simulink model "PhilippePetit_architecture"  (R2020b)
settings: Solver=VariableStepAuto  StartTime=0.0  StopTime=10.0  RelTol=1e-3
settings Model: Creator=nicol  LastModifiedBy=nicol

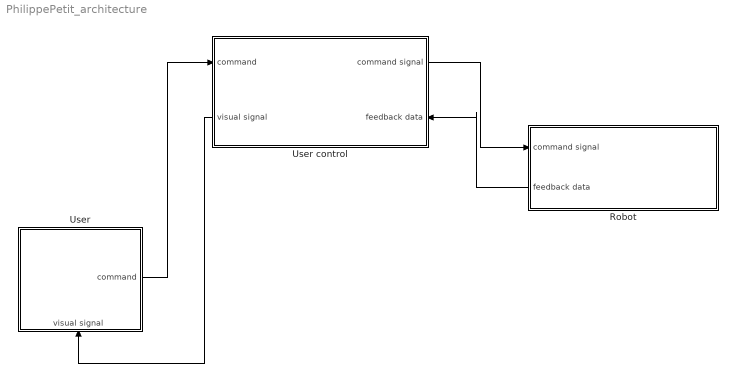
== system PhilippePetit_architecture ==
  Robot : Subsystem
      settings: PortSchema="{\"entries\":[{\"content\":{\"headerSize\":26,\"margin\":15,\"minimumSpacing\":25,\"sides\":[{\"content\":{\"connectorIds\":[\"In1\",\"Out1\"]},\"type\":\"ConnectorPlacement.EquallySpacedRectSide\",\"uuid\":\"a13b1b13-38f4-4b06-bb72-140aa99d31de\"},{\"content\":{\"connectorIds\":[],\"side\":\"RIGHT\"},\"type\":\"ConnectorPlacement.EquallySpacedRectSide\",\"uuid\":\"03928bee-4773-4998-99f8-4502b0986fa4\"},{\"content\":{\"connectorIds\":[],\"side\":\"TOP\"},\"type\":\"ConnectorPlacement.EquallySpacedRectSide\",\"uuid\":\"614edb4f-75a9-4b46-be23-a150b878b705\"},{\"content\":{\"connectorIds\":[],\"side\":\"BOTTOM\"},\"type\":\"ConnectorPlacement.EquallySpacedRectSide\",\"uuid\":\"73503f2b-8796-4b66-885d-2b8b1e679955\"},{\"content\":{\"connectorIds\":[],\"side\":\"HIDDEN\"},\"type\":\"ConnectorPlacement.EquallySpacedRectSide\",\"uuid\":\"9ce51372-9279-48e8-af61-c2921102bc5c\"}]},\"type\":\"ConnectorPlacement.EquallySpacedConnector\",\"uuid\":\"eab28fec-6cb4-4970-8796-7f8236b3d049\"}],\"packageUris\":[\"http://schema.mathworks.com/mf0/Connector/R2020b\"],\"version\":\"1.0\"}"
  User : Subsystem
      settings: PortSchema="{\"entries\":[{\"content\":{\"headerSize\":26,\"margin\":15,\"minimumSpacing\":25,\"sides\":[{\"content\":{\"connectorIds\":[]},\"type\":\"ConnectorPlacement.EquallySpacedRectSide\",\"uuid\":\"fe61efcc-83aa-4783-a816-baaa20b10315\"},{\"content\":{\"connectorIds\":[\"Out1\"],\"side\":\"RIGHT\"},\"type\":\"ConnectorPlacement.EquallySpacedRectSide\",\"uuid\":\"af858a2b-5332-46b9-9432-959710be5434\"},{\"content\":{\"connectorIds\":[],\"side\":\"TOP\"},\"type\":\"ConnectorPlacement.EquallySpacedRectSide\",\"uuid\":\"0d27328e-6c51-4811-958e-b304a9a2605e\"},{\"content\":{\"connectorIds\":[\"In1\"],\"side\":\"BOTTOM\"},\"type\":\"ConnectorPlacement.EquallySpacedRectSide\",\"uuid\":\"966ce028-5962-4a17-8d73-90c152cb0045\"},{\"content\":{\"connectorIds\":[],\"side\":\"HIDDEN\"},\"type\":\"ConnectorPlacement.EquallySpacedRectSide\",\"uuid\":\"1191bd8a-d3b3-41e0-ab93-51888f24952b\"}]},\"type\":\"ConnectorPlacement.EquallySpacedConnector\",\"uuid\":\"d4b5a27a-45d4-44c0-bb5f-ae7473592f44\"}],\"packageUris\":[\"http://schema.mathworks.com/mf0/Connector/R2020b\"],\"version\":\"1.0\"}"
  User control : Subsystem
      settings: PortSchema="{\"entries\":[{\"content\":{\"headerSize\":26,\"margin\":15,\"minimumSpacing\":25,\"sides\":[{\"content\":{\"connectorIds\":[\"In1\",\"Out1\"]},\"type\":\"ConnectorPlacement.EquallySpacedRectSide\",\"uuid\":\"a13b1b13-38f4-4b06-bb72-140aa99d31de\"},{\"content\":{\"connectorIds\":[\"Out2\",\"In2\"],\"side\":\"RIGHT\"},\"type\":\"ConnectorPlacement.EquallySpacedRectSide\",\"uuid\":\"03928bee-4773-4998-99f8-4502b0986fa4\"},{\"content\":{\"connectorIds\":[],\"side\":\"TOP\"},\"type\":\"ConnectorPlacement.EquallySpacedRectSide\",\"uuid\":\"614edb4f-75a9-4b46-be23-a150b878b705\"},{\"content\":{\"connectorIds\":[],\"side\":\"HIDDEN\"},\"type\":\"ConnectorPlacement.EquallySpacedRectSide\",\"uuid\":\"9ce51372-9279-48e8-af61-c2921102bc5c\"}]},\"type\":\"ConnectorPlacement.EquallySpacedConnector\",\"uuid\":\"eab28fec-6cb4-4970-8796-7f8236b3d049\"}],\"packageUris\":[\"http://schema.mathworks.com/mf0/Connector/R2020b\"],\"version\":\"1.0\"}"
  wires:
  User/1(command) -> User control/1(command)
  User control/1(visual signal) -> User/1(visual signal)
  User control/2(command signal) -> Robot/1(" command signal")
  Robot/1(feedback data) -> User control/2(feedback data)

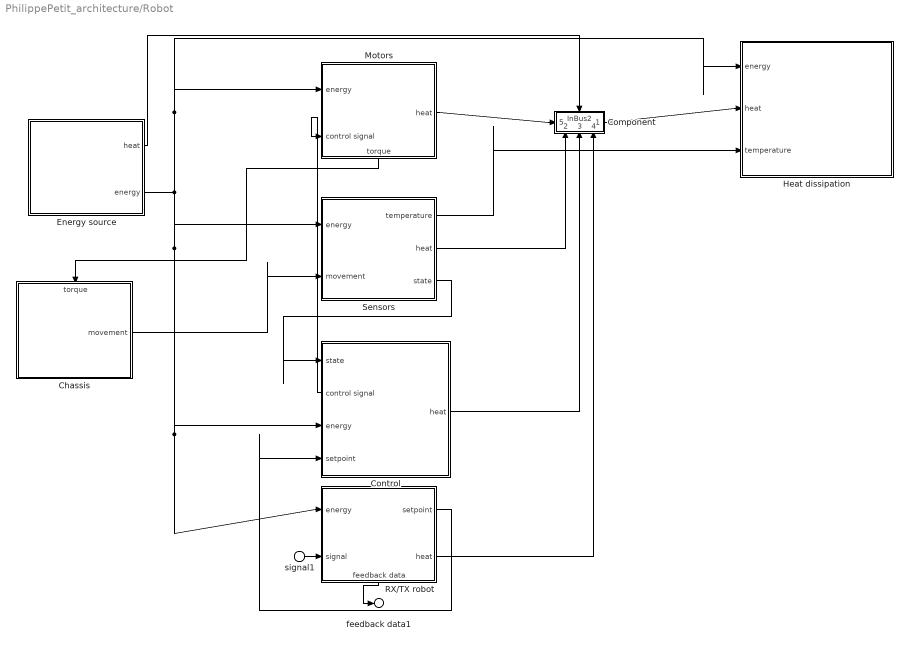
== system PhilippePetit_architecture/Robot ==
  " signal1" : Inport  PortName=command signal
  Chassis : Subsystem
      settings: PortSchema="{\"entries\":[{\"content\":{\"headerSize\":26,\"margin\":15,\"minimumSpacing\":25,\"sides\":[{\"content\":{\"connectorIds\":[]},\"type\":\"ConnectorPlacement.EquallySpacedRectSide\",\"uuid\":\"fe61efcc-83aa-4783-a816-baaa20b10315\"},{\"content\":{\"connectorIds\":[\"Out1\"],\"side\":\"RIGHT\"},\"type\":\"ConnectorPlacement.EquallySpacedRectSide\",\"uuid\":\"af858a2b-5332-46b9-9432-959710be5434\"},{\"content\":{\"connectorIds\":[\"In1\"],\"side\":\"TOP\"},\"type\":\"ConnectorPlacement.EquallySpacedRectSide\",\"uuid\":\"0d27328e-6c51-4811-958e-b304a9a2605e\"},{\"content\":{\"connectorIds\":[],\"side\":\"HIDDEN\"},\"type\":\"ConnectorPlacement.EquallySpacedRectSide\",\"uuid\":\"1191bd8a-d3b3-41e0-ab93-51888f24952b\"}]},\"type\":\"ConnectorPlacement.EquallySpacedConnector\",\"uuid\":\"d4b5a27a-45d4-44c0-bb5f-ae7473592f44\"}],\"packageUris\":[\"http://schema.mathworks.com/mf0/Connector/R2020b\"],\"version\":\"1.0\"}"
  Component : Subsystem
      settings: PortSchema="{\"entries\":[{\"content\":{\"margin\":10,\"minimumSpacing\":15,\"sides\":[{\"content\":{\"connectorIds\":[\"In5\"]},\"type\":\"ConnectorPlacement.EquallySpacedRectSide\",\"uuid\":\"fe61efcc-83aa-4783-a816-baaa20b10315\"},{\"content\":{\"connectorIds\":[\"Out1\"],\"side\":\"RIGHT\"},\"type\":\"ConnectorPlacement.EquallySpacedRectSide\",\"uuid\":\"af858a2b-5332-46b9-9432-959710be5434\"},{\"content\":{\"connectorIds\":[\"In1\"],\"side\":\"TOP\"},\"type\":\"ConnectorPlacement.EquallySpacedRectSide\",\"uuid\":\"0d27328e-6c51-4811-958e-b304a9a2605e\"},{\"content\":{\"connectorIds\":[\"In2\",\"In3\",\"In4\"],\"side\":\"BOTTOM\"},\"type\":\"ConnectorPlacement.EquallySpacedRectSide\",\"uuid\":\"543f712e-d5c5-44b2-9db3-03ae61feada7\"},{\"content\":{\"connectorIds\":[],\"side\":\"HIDDEN\"},\"type\":\"ConnectorPlacement.EquallySpacedRectSide\",\"uuid\":\"1191bd8a-d3b3-41e0-ab93-51888f24952b\"}]},\"type\":\"ConnectorPlacement.EquallySpacedConnector\",\"uuid\":\"d4b5a27a-45d4-44c0-bb5f-ae7473592f44\"}],\"packageUris\":[\"http://schema.mathworks.com/mf0/Connector/R2020b\"],\"version\":\"1.0\"}"
  Control : Subsystem
      settings: PortSchema="{\"entries\":[{\"content\":{\"headerSize\":26,\"margin\":15,\"minimumSpacing\":25,\"sides\":[{\"content\":{\"connectorIds\":[\"In1\",\"Out1\",\"In3\",\"In2\"]},\"type\":\"ConnectorPlacement.EquallySpacedRectSide\",\"uuid\":\"fe61efcc-83aa-4783-a816-baaa20b10315\"},{\"content\":{\"connectorIds\":[\"Out2\"],\"side\":\"RIGHT\"},\"type\":\"ConnectorPlacement.EquallySpacedRectSide\",\"uuid\":\"af858a2b-5332-46b9-9432-959710be5434\"},{\"content\":{\"connectorIds\":[],\"side\":\"TOP\"},\"type\":\"ConnectorPlacement.EquallySpacedRectSide\",\"uuid\":\"0d27328e-6c51-4811-958e-b304a9a2605e\"},{\"content\":{\"connectorIds\":[],\"side\":\"HIDDEN\"},\"type\":\"ConnectorPlacement.EquallySpacedRectSide\",\"uuid\":\"1191bd8a-d3b3-41e0-ab93-51888f24952b\"}]},\"type\":\"ConnectorPlacement.EquallySpacedConnector\",\"uuid\":\"d4b5a27a-45d4-44c0-bb5f-ae7473592f44\"}],\"packageUris\":[\"http://schema.mathworks.com/mf0/Connector/R2020b\"],\"version\":\"1.0\"}"
  Energy source : Subsystem
      settings: PortSchema="{\"entries\":[{\"content\":{\"headerSize\":26,\"margin\":15,\"minimumSpacing\":25,\"sides\":[{\"content\":{\"connectorIds\":[]},\"type\":\"ConnectorPlacement.EquallySpacedRectSide\",\"uuid\":\"fe61efcc-83aa-4783-a816-baaa20b10315\"},{\"content\":{\"connectorIds\":[\"Out1\",\"Out2\"],\"side\":\"RIGHT\"},\"type\":\"ConnectorPlacement.EquallySpacedRectSide\",\"uuid\":\"af858a2b-5332-46b9-9432-959710be5434\"},{\"content\":{\"connectorIds\":[],\"side\":\"TOP\"},\"type\":\"ConnectorPlacement.EquallySpacedRectSide\",\"uuid\":\"0d27328e-6c51-4811-958e-b304a9a2605e\"},{\"content\":{\"connectorIds\":[],\"side\":\"HIDDEN\"},\"type\":\"ConnectorPlacement.EquallySpacedRectSide\",\"uuid\":\"1191bd8a-d3b3-41e0-ab93-51888f24952b\"}]},\"type\":\"ConnectorPlacement.EquallySpacedConnector\",\"uuid\":\"d4b5a27a-45d4-44c0-bb5f-ae7473592f44\"}],\"packageUris\":[\"http://schema.mathworks.com/mf0/Connector/R2020b\"],\"version\":\"1.0\"}"
  Heat dissipation : Subsystem
      settings: PortSchema="{\"entries\":[{\"content\":{\"headerSize\":26,\"margin\":15,\"minimumSpacing\":25,\"sides\":[{\"content\":{\"connectorIds\":[\"In1\",\"In2\",\"In3\"]},\"type\":\"ConnectorPlacement.EquallySpacedRectSide\",\"uuid\":\"fe61efcc-83aa-4783-a816-baaa20b10315\"},{\"content\":{\"connectorIds\":[],\"side\":\"RIGHT\"},\"type\":\"ConnectorPlacement.EquallySpacedRectSide\",\"uuid\":\"af858a2b-5332-46b9-9432-959710be5434\"},{\"content\":{\"connectorIds\":[],\"side\":\"TOP\"},\"type\":\"ConnectorPlacement.EquallySpacedRectSide\",\"uuid\":\"0d27328e-6c51-4811-958e-b304a9a2605e\"},{\"content\":{\"connectorIds\":[],\"side\":\"HIDDEN\"},\"type\":\"ConnectorPlacement.EquallySpacedRectSide\",\"uuid\":\"1191bd8a-d3b3-41e0-ab93-51888f24952b\"}]},\"type\":\"ConnectorPlacement.EquallySpacedConnector\",\"uuid\":\"d4b5a27a-45d4-44c0-bb5f-ae7473592f44\"}],\"packageUris\":[\"http://schema.mathworks.com/mf0/Connector/R2020b\"],\"version\":\"1.0\"}"
  Motors : Subsystem
      settings: PortSchema="{\"entries\":[{\"content\":{\"headerSize\":26,\"margin\":15,\"minimumSpacing\":25,\"sides\":[{\"content\":{\"connectorIds\":[\"In1\",\"In2\"]},\"type\":\"ConnectorPlacement.EquallySpacedRectSide\",\"uuid\":\"fe61efcc-83aa-4783-a816-baaa20b10315\"},{\"content\":{\"connectorIds\":[\"Out2\"],\"side\":\"RIGHT\"},\"type\":\"ConnectorPlacement.EquallySpacedRectSide\",\"uuid\":\"af858a2b-5332-46b9-9432-959710be5434\"},{\"content\":{\"connectorIds\":[],\"side\":\"TOP\"},\"type\":\"ConnectorPlacement.EquallySpacedRectSide\",\"uuid\":\"0d27328e-6c51-4811-958e-b304a9a2605e\"},{\"content\":{\"connectorIds\":[\"Out1\"],\"side\":\"BOTTOM\"},\"type\":\"ConnectorPlacement.EquallySpacedRectSide\",\"uuid\":\"ab8045d5-2f64-4f7d-896e-5133e5fbee7e\"},{\"content\":{\"connectorIds\":[],\"side\":\"HIDDEN\"},\"type\":\"ConnectorPlacement.EquallySpacedRectSide\",\"uuid\":\"1191bd8a-d3b3-41e0-ab93-51888f24952b\"}]},\"type\":\"ConnectorPlacement.EquallySpacedConnector\",\"uuid\":\"d4b5a27a-45d4-44c0-bb5f-ae7473592f44\"}],\"packageUris\":[\"http://schema.mathworks.com/mf0/Connector/R2020b\"],\"version\":\"1.0\"}"
  RX/TX robot : Subsystem
      settings: PortSchema="{\"entries\":[{\"content\":{\"headerSize\":26,\"margin\":15,\"minimumSpacing\":25,\"sides\":[{\"content\":{\"connectorIds\":[\"In2\",\"In1\"]},\"type\":\"ConnectorPlacement.EquallySpacedRectSide\",\"uuid\":\"fe61efcc-83aa-4783-a816-baaa20b10315\"},{\"content\":{\"connectorIds\":[\"Out2\",\"Out3\"],\"side\":\"RIGHT\"},\"type\":\"ConnectorPlacement.EquallySpacedRectSide\",\"uuid\":\"af858a2b-5332-46b9-9432-959710be5434\"},{\"content\":{\"connectorIds\":[],\"side\":\"TOP\"},\"type\":\"ConnectorPlacement.EquallySpacedRectSide\",\"uuid\":\"0d27328e-6c51-4811-958e-b304a9a2605e\"},{\"content\":{\"connectorIds\":[\"Out1\"],\"side\":\"BOTTOM\"},\"type\":\"ConnectorPlacement.EquallySpacedRectSide\",\"uuid\":\"3b3053d7-3574-47a1-96ff-38e328b25c8b\"},{\"content\":{\"connectorIds\":[],\"side\":\"HIDDEN\"},\"type\":\"ConnectorPlacement.EquallySpacedRectSide\",\"uuid\":\"1191bd8a-d3b3-41e0-ab93-51888f24952b\"}]},\"type\":\"ConnectorPlacement.EquallySpacedConnector\",\"uuid\":\"d4b5a27a-45d4-44c0-bb5f-ae7473592f44\"}],\"packageUris\":[\"http://schema.mathworks.com/mf0/Connector/R2020b\"],\"version\":\"1.0\"}"
  Sensors : Subsystem
      settings: PortSchema="{\"entries\":[{\"content\":{\"headerSize\":26,\"margin\":15,\"minimumSpacing\":25,\"sides\":[{\"content\":{\"connectorIds\":[\"In1\",\"In2\"]},\"type\":\"ConnectorPlacement.EquallySpacedRectSide\",\"uuid\":\"fe61efcc-83aa-4783-a816-baaa20b10315\"},{\"content\":{\"connectorIds\":[\"Out1\",\"Out2\",\"Out3\"],\"side\":\"RIGHT\"},\"type\":\"ConnectorPlacement.EquallySpacedRectSide\",\"uuid\":\"af858a2b-5332-46b9-9432-959710be5434\"},{\"content\":{\"connectorIds\":[],\"side\":\"TOP\"},\"type\":\"ConnectorPlacement.EquallySpacedRectSide\",\"uuid\":\"0d27328e-6c51-4811-958e-b304a9a2605e\"},{\"content\":{\"connectorIds\":[],\"side\":\"HIDDEN\"},\"type\":\"ConnectorPlacement.EquallySpacedRectSide\",\"uuid\":\"1191bd8a-d3b3-41e0-ab93-51888f24952b\"}]},\"type\":\"ConnectorPlacement.EquallySpacedConnector\",\"uuid\":\"d4b5a27a-45d4-44c0-bb5f-ae7473592f44\"}],\"packageUris\":[\"http://schema.mathworks.com/mf0/Connector/R2020b\"],\"version\":\"1.0\"}"
  feedback data1 : Outport  PortName=feedback data
  wires:
  Control/2(heat) -> Component/3(InBus1)
  Energy source/2(energy) -> Heat dissipation/1(energy), Motors/1(energy), RX/TX robot/2(energy), Control/3(energy), Sensors/1(energy)
  Sensors/2(heat) -> Component/2(InBus)
  Sensors/3(state) -> Control/1(state)
  Sensors/1(temperature) -> Heat dissipation/3(temperature)
  RX/TX robot/1(feedback data) -> feedback data1/1
  RX/TX robot/2(setpoint) -> Control/2(setpoint)
  Component/1(tot heat) -> Heat dissipation/2(heat)
  RX/TX robot/3(heat) -> Component/4(heat)
  Motors/2(heat) -> Component/5(heat1)
  " signal1"/1 -> RX/TX robot/1(" signal")
  Energy source/1(heat) -> Component/1(InBus2)
  Control/1(control signal) -> Motors/2(control signal)
  Motors/1(torque) -> Chassis/1(torque)
  Chassis/1(movement) -> Sensors/2(movement)

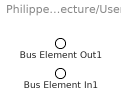
== system PhilippePetit_architecture/User ==
  Bus Element In1 : Inport  PortName=visual signal
  Bus Element Out1 : Outport  PortName=command

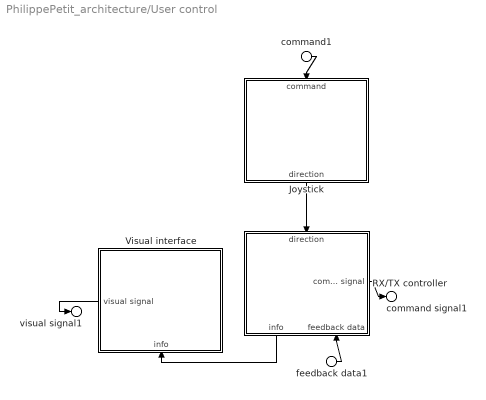
== system PhilippePetit_architecture/User control ==
  command1 : Inport  PortName=command
  feedback data1 : Inport  Port=2  PortName=feedback data
  Joystick : Subsystem
      settings: PortSchema="{\"entries\":[{\"content\":{\"headerSize\":26,\"margin\":15,\"minimumSpacing\":25,\"sides\":[{\"content\":{\"connectorIds\":[]},\"type\":\"ConnectorPlacement.EquallySpacedRectSide\",\"uuid\":\"fe61efcc-83aa-4783-a816-baaa20b10315\"},{\"content\":{\"connectorIds\":[],\"side\":\"RIGHT\"},\"type\":\"ConnectorPlacement.EquallySpacedRectSide\",\"uuid\":\"af858a2b-5332-46b9-9432-959710be5434\"},{\"content\":{\"connectorIds\":[\"In1\"],\"side\":\"TOP\"},\"type\":\"ConnectorPlacement.EquallySpacedRectSide\",\"uuid\":\"0d27328e-6c51-4811-958e-b304a9a2605e\"},{\"content\":{\"connectorIds\":[\"Out1\"],\"side\":\"BOTTOM\"},\"type\":\"ConnectorPlacement.EquallySpacedRectSide\",\"uuid\":\"2fc8f7ae-d563-416e-94db-7c5ffa9122e4\"},{\"content\":{\"connectorIds\":[],\"side\":\"HIDDEN\"},\"type\":\"ConnectorPlacement.EquallySpacedRectSide\",\"uuid\":\"1191bd8a-d3b3-41e0-ab93-51888f24952b\"}]},\"type\":\"ConnectorPlacement.EquallySpacedConnector\",\"uuid\":\"d4b5a27a-45d4-44c0-bb5f-ae7473592f44\"}],\"packageUris\":[\"http://schema.mathworks.com/mf0/Connector/R2020b\"],\"version\":\"1.0\"}"
  RX/TX controller : Subsystem
      settings: PortSchema="{\"entries\":[{\"content\":{\"headerSize\":26,\"margin\":15,\"minimumSpacing\":25,\"sides\":[{\"content\":{\"connectorIds\":[]},\"type\":\"ConnectorPlacement.EquallySpacedRectSide\",\"uuid\":\"fe61efcc-83aa-4783-a816-baaa20b10315\"},{\"content\":{\"connectorIds\":[\"Out2\"],\"side\":\"RIGHT\"},\"type\":\"ConnectorPlacement.EquallySpacedRectSide\",\"uuid\":\"af858a2b-5332-46b9-9432-959710be5434\"},{\"content\":{\"connectorIds\":[\"In2\"],\"side\":\"TOP\"},\"type\":\"ConnectorPlacement.EquallySpacedRectSide\",\"uuid\":\"0d27328e-6c51-4811-958e-b304a9a2605e\"},{\"content\":{\"connectorIds\":[\"Out1\",\"In1\"],\"side\":\"BOTTOM\"},\"type\":\"ConnectorPlacement.EquallySpacedRectSide\",\"uuid\":\"e34f4db2-095e-4c46-8f72-d51fa938d794\"},{\"content\":{\"connectorIds\":[],\"side\":\"HIDDEN\"},\"type\":\"ConnectorPlacement.EquallySpacedRectSide\",\"uuid\":\"1191bd8a-d3b3-41e0-ab93-51888f24952b\"}]},\"type\":\"ConnectorPlacement.EquallySpacedConnector\",\"uuid\":\"d4b5a27a-45d4-44c0-bb5f-ae7473592f44\"}],\"packageUris\":[\"http://schema.mathworks.com/mf0/Connector/R2020b\"],\"version\":\"1.0\"}"
  Visual interface : Subsystem
      settings: PortSchema="{\"entries\":[{\"content\":{\"headerSize\":26,\"margin\":15,\"minimumSpacing\":25,\"sides\":[{\"content\":{\"connectorIds\":[\"Out1\"]},\"type\":\"ConnectorPlacement.EquallySpacedRectSide\",\"uuid\":\"fe61efcc-83aa-4783-a816-baaa20b10315\"},{\"content\":{\"connectorIds\":[],\"side\":\"RIGHT\"},\"type\":\"ConnectorPlacement.EquallySpacedRectSide\",\"uuid\":\"af858a2b-5332-46b9-9432-959710be5434\"},{\"content\":{\"connectorIds\":[],\"side\":\"TOP\"},\"type\":\"ConnectorPlacement.EquallySpacedRectSide\",\"uuid\":\"0d27328e-6c51-4811-958e-b304a9a2605e\"},{\"content\":{\"connectorIds\":[\"In1\"],\"side\":\"BOTTOM\"},\"type\":\"ConnectorPlacement.EquallySpacedRectSide\",\"uuid\":\"5a0afe0c-1d89-46be-b1ab-40f5f276f1ed\"},{\"content\":{\"connectorIds\":[],\"side\":\"HIDDEN\"},\"type\":\"ConnectorPlacement.EquallySpacedRectSide\",\"uuid\":\"1191bd8a-d3b3-41e0-ab93-51888f24952b\"}]},\"type\":\"ConnectorPlacement.EquallySpacedConnector\",\"uuid\":\"d4b5a27a-45d4-44c0-bb5f-ae7473592f44\"}],\"packageUris\":[\"http://schema.mathworks.com/mf0/Connector/R2020b\"],\"version\":\"1.0\"}"
  visual signal1 : Outport  PortName=visual signal
  command signal1 : Outport  Port=2  PortName=command signal
  wires:
  RX/TX controller/2(command signal) -> command signal1/1
  Joystick/1(direction) -> RX/TX controller/2(direction)
  feedback data1/1 -> RX/TX controller/1(feedback data)
  command1/1 -> Joystick/1(command)
  RX/TX controller/1(info) -> Visual interface/1(info)
  Visual interface/1(visual signal) -> visual signal1/1

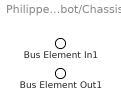
== system PhilippePetit_architecture/Robot/Chassis ==
  Bus Element In1 : Inport  PortName=torque
  Bus Element Out1 : Outport  PortName=movement

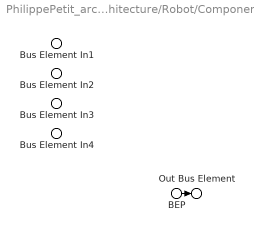
== system PhilippePetit_architecture/Robot/Component ==
  Bus Element In4 : Inport  PortName=InBus2
  Bus Element In2 : Inport  Port=2  PortName=InBus
  Bus Element In3 : Inport  Port=3  PortName=InBus1
  Bus Element In1 : Inport  Port=4  PortName=heat
  BEP : Inport  Port=5  PortName=heat1
  Out Bus Element : Outport  PortName=tot heat
  wires:
  BEP/1 -> Out Bus Element/1

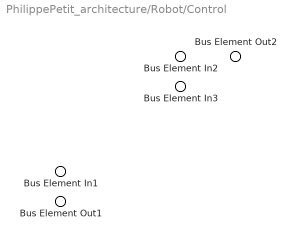
== system PhilippePetit_architecture/Robot/Control ==
  Bus Element In3 : Inport  PortName=state
  Bus Element In2 : Inport  Port=2  PortName=setpoint
  Bus Element In1 : Inport  Port=3  PortName=energy
  Bus Element Out2 : Outport  PortName=control signal
  Bus Element Out1 : Outport  Port=2  PortName=heat

== system PhilippePetit_architecture/Robot/Energy source ==
  Bus Element Out2 : Outport  PortName=heat
  Bus Element Out1 : Outport  Port=2  PortName=energy

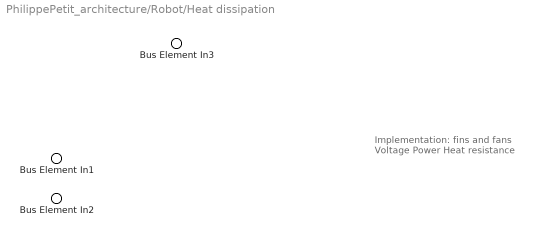
== system PhilippePetit_architecture/Robot/Heat dissipation ==
  note: Implementation: fins and fans
      | Voltage
      | Power
      | Heat resistance
  Bus Element In3 : Inport  PortName=energy
  Bus Element In1 : Inport  Port=2  PortName=heat
  Bus Element In2 : Inport  Port=3  PortName=temperature

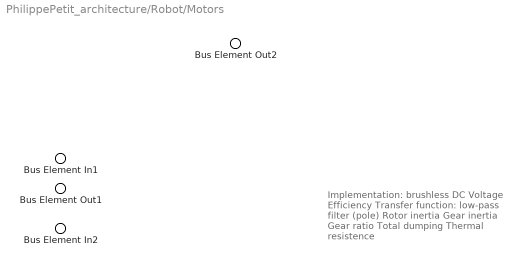
== system PhilippePetit_architecture/Robot/Motors ==
  note: Implementation: brushless DC
      | Voltage
      | Efficiency
      | Transfer function: low-pass filter (pole)
      | Rotor inertia
      | Gear inertia
      | Gear ratio
      | Total dumping
      | Thermal resistence
  Bus Element In1 : Inport  PortName=energy
  Bus Element In2 : Inport  Port=2  PortName=control signal
  Bus Element Out2 : Outport  PortName=torque
  Bus Element Out1 : Outport  Port=2  PortName=heat

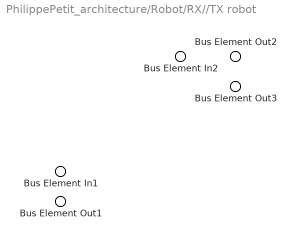
== system PhilippePetit_architecture/Robot/RX//TX robot ==
  Bus Element In2 : Inport  PortName=signal
  Bus Element In1 : Inport  Port=2  PortName=energy
  Bus Element Out3 : Outport  PortName=feedback data
  Bus Element Out2 : Outport  Port=2  PortName=setpoint
  Bus Element Out1 : Outport  Port=3  PortName=heat

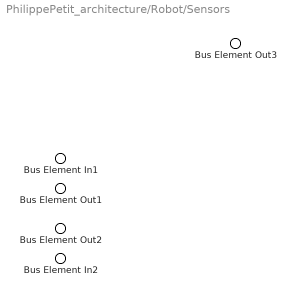
== system PhilippePetit_architecture/Robot/Sensors ==
  Bus Element In1 : Inport  PortName=energy
  Bus Element In2 : Inport  Port=2  PortName=movement
  Bus Element Out3 : Outport  PortName=temperature
  Bus Element Out1 : Outport  Port=2  PortName=heat
  Bus Element Out2 : Outport  Port=3  PortName=state

== system PhilippePetit_architecture/User control/Joystick ==
  Bus Element In1 : Inport  PortName=command
  Bus Element Out1 : Outport  PortName=direction

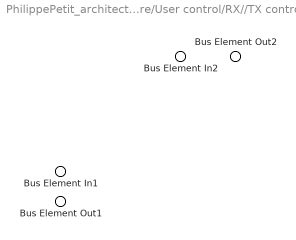
== system PhilippePetit_architecture/User control/RX//TX controller ==
  Bus Element In2 : Inport  PortName=feedback data
  Bus Element In1 : Inport  Port=2  PortName=direction
  Bus Element Out2 : Outport  PortName=info
  Bus Element Out1 : Outport  Port=2  PortName=command signal

== system PhilippePetit_architecture/User control/Visual interface ==
  Bus Element In1 : Inport  PortName=info
  Bus Element Out1 : Outport  PortName=visual signal
